simulink model "LFR_Simulink"  (R2024a)
settings: Solver=FixedStepDiscrete  StartTime=0.0  StopTime=inf  FixedStep=0.01  RelTol=1e-3
undefined symbols (not defined in the file or in its folder): motorIp, motorSp
libraries: mobileRoboticsTrainingLib x5
settings Model: Creator=IT5  LastModifiedBy=IT5

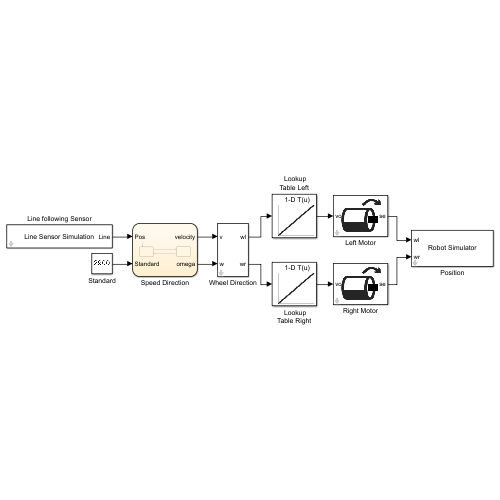
[thumbnail: Simulink's stored preview of the top-level diagram]
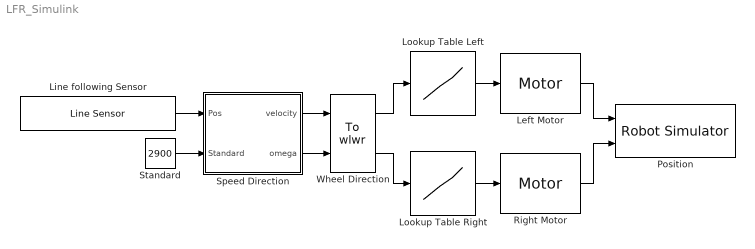
== system LFR_Simulink ==
  " Lookup Table Left" : Lookup_n-D  NumberOfTableDimensions=1  BreakpointsForDimension1=motorSp  Table=motorIp  ExtrapMethod=Clip  InternalRulePriority=Speed  RndMeth=Simplest
  " Lookup Table Right" : Lookup_n-D  NumberOfTableDimensions=1  BreakpointsForDimension1=motorSp  Table=motorIp  ExtrapMethod=Clip  InternalRulePriority=Speed  RndMeth=Simplest
  Left Motor : mobileRoboticsTrainingLib/Motor  motorPlant=wheelMotorModel  sensorType=Speed
      settings: SourceProductName=Mobile Robotics Training Library
  Line following Sensor : mobileRoboticsTrainingLib/Line Sensor  mapVariable=mapForSim  envVal=2850  lineVal=2950  sensOff=[0.01 0]
      settings: SourceProductName=Mobile Robotics Training Library
  Position : mobileRoboticsTrainingLib/Robot Simulator  Priority=99  mapVar=mapForSim  startX=0.39401  startY=1.4914  startTheta=0  axleLength=axleLength  wheelR=wheelR
  Right Motor : mobileRoboticsTrainingLib/Motor  motorPlant=wheelMotorModel  sensorType=Speed
      settings: SourceProductName=Mobile Robotics Training Library
  Speed Direction : Stateflow chart  TreatAsAtomicUnit=on
  Standard : Constant  Value=2900
  Wheel Direction : mobileRoboticsTrainingLib/To wlwr  axleLength=axleLength  wheelR=wheelR
  wires:
  Standard/1 -> Speed Direction/2(Standard)
  Line following Sensor/1 -> Speed Direction/1(Pos)
  Speed Direction/2(omega) -> Wheel Direction/2
  Speed Direction/1(velocity) -> Wheel Direction/1
  Left Motor/1 -> Position/1
  Right Motor/1 -> Position/2
  " Lookup Table Left"/1 -> Left Motor/1
  Wheel Direction/1 -> " Lookup Table Left"/1
  " Lookup Table Right"/1 -> Right Motor/1
  Wheel Direction/2 -> " Lookup Table Right"/1

== stateflow chart LFR_Simulink/Speed Direction ==
  state RightSide
    velocity =0.05;
    omega = -1;
  state LeftSide
    velocity =0.05;
    omega = 1;
  (default) -> LeftSide
  LeftSide -> RightSide : [Pos < Standard]
  RightSide -> LeftSide : [Pos >= Standard]
  data: Pos input; Standard input; velocity output; omega output
